simulink model "controller14"  (R2023a)
settings: Solver=FixedStepAuto  StartTime=0.0  StopTime=mdl.rt  RelTol=1e-3
values from neighbouring files (symbols this model uses):
  ctr = make_ext_tor_observer(rsim, mdl, ctr)    [step1_setup.m]
  ctr2 = ctr    [step1_setup.m]
  mdl = make_model(mdl,rsim)    [step1_setup.m]
  rbt = make_robot    [step1_setup.m]
  rbt2 = rbt    [step1_setup.m]
  som = make_somersault(mdl, rsim)    [step1_setup.m]
  traj = make_trajectory(ctr, mdl, rsim)    [step1_setup.m]
undefined symbols (not defined in the file or in its folder): archived_Eul_XYZ, archived_p_raw, DiscIntNeverNeededParam, lut, rsim, Standard_Devices, UDP_Protocol
libraries: simulink x27, dspfdesign x7, robotcorelib x6, sldrtlib x4, slrealtimeloglib x1, shared6dof x1, dspsrcs4 x1, uavutilslib x1
(part 2 of 3)

== system controller14/State filters/Subsystem1 ==
  p_dot : Inport
  data ready : Inport  Port=2
  Add1 : Sum  Inputs=+-
  Add2 : Sum  Inputs=+-
  Add3 : Sum  Commented=on  Inputs=+-
  Add4 : Sum  Inputs=+-
  Delay : Delay  Commented=on  DelayLength=1  InitialCondition=zeros(3,1)
  Delay1 : Delay  DelayLength=1  InitialCondition=zeros(3,1)
  Digital Filter Design2 : dspfdesign/Digital Filter Design  Commented=on  mwdsp_browser_bugfix_var=off
  Digital Clock : DigitalClock  SampleTime=mdl.T_high
  Gain : Gain  Commented=on  Gain=mdl.f_high
  Gain1 : Gain  Gain=mdl.f_high
  If : If  IfExpression=u1 == 0
  If Action Subsystem : Subsystem  TreatAsAtomicUnit=on
  If Action Subsystem1 : Subsystem  TreatAsAtomicUnit=on
  Merge : Merge
  Scope : Scope  Commented=on  NumInputPorts=2
  Triggered Subsystem : Subsystem  TreatAsAtomicUnit=on
  p_dotdot : Outport
  wires:
  data ready/1 -> Triggered Subsystem/Trigger
  Triggered Subsystem/1(Out1) -> Add1/1
  Triggered Subsystem/2(Output) -> Add1/2
  Triggered Subsystem/3(Output1) -> Add2/1
  Triggered Subsystem/4(Output2) -> Add2/2
  Add1/1 -> If Action Subsystem/1(In1)
  Add2/1 -> If Action Subsystem/2(In2), If/1
  If/2 -> If Action Subsystem/Action
  If/1 -> If Action Subsystem1/Action
  If Action Subsystem1/1(Out1) -> Merge/2
  If Action Subsystem/1(Out1) -> Merge/1
  Digital Clock/1 -> Triggered Subsystem/2(In2)
  Digital Filter Design2/1 -> Delay/1, Add3/1  "p_dot_filtered"
  Delay/1 -> Add3/2
  Add3/1 -> Gain/1
  Gain/1 -> Scope/2
  Add4/1 -> Gain1/1
  Delay1/1 -> Add4/2
  p_dot/1 -> Delay1/1, Add4/1, Digital Filter Design2/1, Triggered Subsystem/1(In1)  "p_dot_filtered"
  Gain1/1 -> p_dotdot/1, Scope/1

== system controller14/State filters/Subsystem4 ==
  In1 : Inport
  data ready : Inport  Port=2
  Add1 : Sum  Inputs=+-
  Add2 : Sum  Inputs=+-
  Digital Filter Design1 : dspfdesign/Digital Filter Design  mwdsp_browser_bugfix_var=off
  Digital Filter Design2 : dspfdesign/Digital Filter Design  Commented=on  mwdsp_browser_bugfix_var=off
  Digital Clock : DigitalClock  SampleTime=mdl.T_high
  If : If  IfExpression=u1 == 0
  If Action Subsystem : Subsystem  TreatAsAtomicUnit=on
  If Action Subsystem1 : Subsystem  TreatAsAtomicUnit=on
  Merge : Merge
  Scope : Scope  Commented=on  NumInputPorts=2
  Triggered Subsystem : Subsystem  TreatAsAtomicUnit=on
  p dot : Outport
  wires:
  In1/1 -> Triggered Subsystem/1(In1)
  data ready/1 -> Triggered Subsystem/Trigger
  Triggered Subsystem/1(Out1) -> Add1/1
  Triggered Subsystem/2(Output) -> Add1/2
  Triggered Subsystem/3(Output1) -> Add2/1
  Triggered Subsystem/4(Output2) -> Add2/2
  Add1/1 -> If Action Subsystem/1(In1)
  Add2/1 -> If Action Subsystem/2(In2), If/1
  If/2 -> If Action Subsystem/Action
  If/1 -> If Action Subsystem1/Action
  If Action Subsystem1/1(Out1) -> Merge/2
  If Action Subsystem/1(Out1) -> Merge/1
  Merge/1 -> Digital Filter Design1/1, Scope/1
  Digital Clock/1 -> Triggered Subsystem/2(In2)
  Digital Filter Design1/1 -> Scope/2, p dot/1  "p_dot_filtered"

== system controller14/State filters/Subsystem5 ==
  euler_angles : Inport
  data ready : Inport  Port=2
  sim enable : Inport  Port=3
  Add1 : Sum  Inputs=+-
  Add2 : Sum  Inputs=+-
  Add3 : Sum  Inputs=+-
  Delay : Delay  DelayLength=1  InitialCondition=zeros(9,1)
  Digital Clock : DigitalClock  SampleTime=1/10000
  Gain : Gain  Gain=400
  If : If  IfExpression=u1 == 0
  If Action Subsystem : Subsystem  TreatAsAtomicUnit=on
  If Action Subsystem1 : Subsystem  TreatAsAtomicUnit=on
  Merge : Merge
  Rotation Matrix : MATLAB Function  TreatAsAtomicUnit=on
  Rotation Matrix2 : MATLAB Function  TreatAsAtomicUnit=on
  Rotation Matrix3 : MATLAB Function  TreatAsAtomicUnit=on
  Switch1 : Switch  Criteria=u2 > Threshold  SaturateOnIntegerOverflow=off  InputSameDT=off
  Switch2 : Switch  Criteria=u2 > Threshold  SaturateOnIntegerOverflow=off  InputSameDT=off
  Triggered Subsystem : Subsystem  TreatAsAtomicUnit=on
  R : Outport
  Rdot : Outport  Port=2
  Omega : Outport  Port=3
  wires:
  Triggered Subsystem/1(Out1) -> Add1/1
  Triggered Subsystem/3(Output1) -> Add2/1
  Triggered Subsystem/4(Output2) -> Add2/2
  If Action Subsystem1/1(Out1) -> Merge/2
  If Action Subsystem/1(Out1) -> Merge/1
  Triggered Subsystem/2(Output) -> Add1/2
  Digital Clock/1 -> Triggered Subsystem/2(In2)
  data ready/1 -> Triggered Subsystem/Trigger
  Add2/1 -> If Action Subsystem/2(In2), If/1
  If/2 -> If Action Subsystem/Action
  If/1 -> If Action Subsystem1/Action
  Add1/1 -> If Action Subsystem/1(In1)
  euler_angles/1 -> Rotation Matrix/1(euler_angles)
  Rotation Matrix/1(R) -> Triggered Subsystem/1(R), R/1, Rotation Matrix3/1(R), Rotation Matrix2/1(R), Delay/1, Add3/1
  Delay/1 -> Add3/2
  Add3/1 -> Gain/1
  sim enable/1 -> Switch2/2, Switch1/2
  Gain/1 -> Switch2/1, Rotation Matrix2/2(Rdot)
  Rotation Matrix2/1(w) -> Switch1/1  "sim_omega"
  Merge/1 -> Switch2/3, Rotation Matrix3/2(Rdot)
  Rotation Matrix3/1(w) -> Switch1/3  "Vicon_omega"
  Switch1/1 -> Omega/1  "p_raw"
  Switch2/1 -> Rdot/1  "p_raw"

== system controller14/Subsystem/time ==
  constant : Constant
  time : DiscreteIntegrator  gainval=1  SampleTime=-1  UpperSaturationLimit=1  LowerSaturationLimit=0  ICPrevOutput=DiscIntNeverNeededParam  ICPrevScaledInput=DiscIntNeverNeededParam
  real times : Outport
  wires:
  constant/1 -> time/1
  time/1 -> real times/1

== system controller14/UDP send to Arduino/UDP send to Arduino DAC ==
  note: Aptinex DAC 20230818
  DAC1 : Inport
  DAC2 : Inport  Port=2
  DAC3 : Inport  Port=3
  DAC4 : Inport  Port=4
  DO2 : Inport  Port=5  OutDataTypeStr=boolean
  Bit Set : simulink/Logic and Bit Operations/Bit Set  iBit=12
  Demux : Demux
  Gain{,1..3} (4 alike) : Gain  Gain=4095/10  OutDataTypeStr=uint16
  Mux : Mux
  Mux1 : Mux
  Saturation : Saturate  UpperLimit=10  LowerLimit=0
  Switch : Switch  Criteria=u2 ~= 0  OutDataTypeStr=uint16  SaturateOnIntegerOverflow=off  InputSameDT=off
  Output : Outport
  wires:
  Gain3/1 -> Mux1/4  "UDP uint16 4"
  Gain1/1 -> Mux1/2  "UDP uint16 2"
  Gain/1 -> Bit Set/1, Switch/3  "UDP uint16 1"
  Gain2/1 -> Mux1/3  "UDP uint16 3"
  DO2/1 -> Switch/2
  Bit Set/1 -> Switch/1
  Mux1/1 -> Output/1
  Switch/1 -> Mux1/1
  Demux/1 -> Gain/1
  Demux/2 -> Gain1/1
  Demux/3 -> Gain2/1
  Demux/4 -> Gain3/1
  DAC1/1 -> Mux/1  "DAC voltage 1"
  DAC2/1 -> Mux/2  "DAC voltage 2"
  DAC3/1 -> Mux/3  "DAC voltage 3"
  DAC4/1 -> Mux/4  "DAC voltage 4"
  Mux/1 -> Saturation/1
  Saturation/1 -> Demux/1

== system controller14/signal generator1/Bias_Signal ==
  note: time constant = 0.002sec
  QuasiEnable : Inport
  BiasVolts : Inport  Port=2
  AveragedBias : Subsystem
  PreGain : Gain
  Product : Product  RndMeth=Zero
  SIgnalForRamp_binary : Subsystem
  SaturatingRamp : DiscreteIntegrator  gainval=100  SampleTime=-1  LimitOutput=on  UpperSaturationLimit=1  LowerSaturationLimit=0  ICPrevOutput=DiscIntNeverNeededParam  ICPrevScaledInput=DiscIntNeverNeededParam
  BiasD2A : Outport
  wires:
  PreGain/1 -> BiasD2A/1
  BiasVolts/1 -> AveragedBias/1(In1)
  QuasiEnable/1 -> SIgnalForRamp_binary/1(In1)
  SIgnalForRamp_binary/1(Out1) -> SaturatingRamp/1
  SaturatingRamp/1 -> Product/1
  AveragedBias/1(Out1) -> Product/2
  Product/1 -> PreGain/1

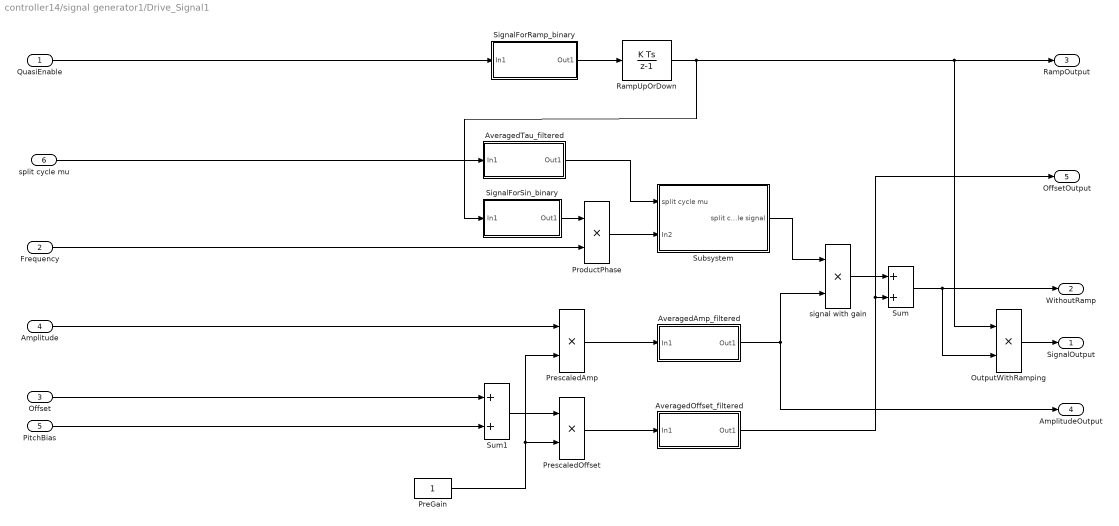
== system controller14/signal generator1/Drive_Signal1 ==
  QuasiEnable : Inport
  Frequency : Inport  Port=2
  Offset : Inport  Port=3
  Amplitude : Inport  Port=4
  PitchBias : Inport  Port=5
  split cycle mu : Inport  Port=6
  AveragedAmp_filtered : Subsystem
  AveragedOffset_filtered : Subsystem
  AveragedTau_filtered : Subsystem
  OutputWithRamping : Product  RndMeth=Zero
  PreGain : Constant
  PrescaledAmp : Product  RndMeth=Zero
  PrescaledOffset : Product  RndMeth=Zero
  ProductPhase : Product  RndMeth=Zero
  RampUpOrDown : DiscreteIntegrator  gainval=100  SampleTime=-1  LimitOutput=on  UpperSaturationLimit=1  LowerSaturationLimit=0  ICPrevOutput=DiscIntNeverNeededParam  ICPrevScaledInput=DiscIntNeverNeededParam
  SignalForRamp_binary : Subsystem
  SignalForSin_binary : Subsystem
  Subsystem : Subsystem
  Sum : Sum
  Sum1 : Sum
  signal with gain : Product  RndMeth=Zero
  SignalOutput : Outport
  WithoutRamp : Outport  Port=2
  RampOutput : Outport  Port=3
  AmplitudeOutput : Outport  Port=4
  OffsetOutput : Outport  Port=5
  wires:
  PrescaledAmp/1 -> AveragedAmp_filtered/1(In1)
  Sum/1 -> OutputWithRamping/2, WithoutRamp/1
  RampUpOrDown/1 -> RampOutput/1, OutputWithRamping/1, SignalForSin_binary/1(In1)
  QuasiEnable/1 -> SignalForRamp_binary/1(In1)
  SignalForRamp_binary/1(Out1) -> RampUpOrDown/1
  Amplitude/1 -> PrescaledAmp/1
  signal with gain/1 -> Sum/1
  Frequency/1 -> ProductPhase/2
  SignalForSin_binary/1(Out1) -> ProductPhase/1
  ProductPhase/1 -> Subsystem/2(In2)
  AveragedOffset_filtered/1(Out1) -> Sum/2, OffsetOutput/1
  PrescaledOffset/1 -> AveragedOffset_filtered/1(In1)
  PreGain/1 -> PrescaledAmp/2, PrescaledOffset/2
  OutputWithRamping/1 -> SignalOutput/1
  AveragedAmp_filtered/1(Out1) -> signal with gain/2, AmplitudeOutput/1
  Sum1/1 -> PrescaledOffset/1
  Offset/1 -> Sum1/1
  PitchBias/1 -> Sum1/2
  AveragedTau_filtered/1(Out1) -> Subsystem/1(split cycle mu)
  split cycle mu/1 -> AveragedTau_filtered/1(In1)
  Subsystem/1(split cycle signal) -> signal with gain/1

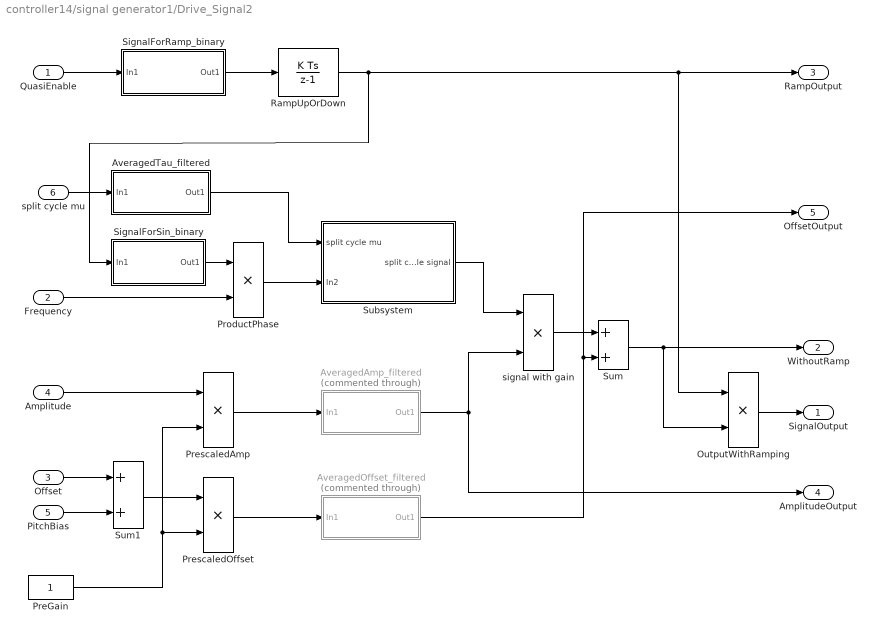
== system controller14/signal generator1/Drive_Signal2 ==
  QuasiEnable : Inport
  Frequency : Inport  Port=2
  Offset : Inport  Port=3
  Amplitude : Inport  Port=4
  PitchBias : Inport  Port=5
  split cycle mu : Inport  Port=6
  AveragedAmp_filtered : Subsystem  Commented=through
  AveragedOffset_filtered : Subsystem  Commented=through
  AveragedTau_filtered : Subsystem
  OutputWithRamping : Product  RndMeth=Zero
  PreGain : Constant
  PrescaledAmp : Product  RndMeth=Zero
  PrescaledOffset : Product  RndMeth=Zero
  ProductPhase : Product  RndMeth=Zero
  RampUpOrDown : DiscreteIntegrator  gainval=100  SampleTime=-1  LimitOutput=on  UpperSaturationLimit=1  LowerSaturationLimit=0  ICPrevOutput=DiscIntNeverNeededParam  ICPrevScaledInput=DiscIntNeverNeededParam
  SignalForRamp_binary : Subsystem
  SignalForSin_binary : Subsystem
  Subsystem : Subsystem
  Sum : Sum
  Sum1 : Sum
  signal with gain : Product  RndMeth=Zero
  SignalOutput : Outport
  WithoutRamp : Outport  Port=2
  RampOutput : Outport  Port=3
  AmplitudeOutput : Outport  Port=4
  OffsetOutput : Outport  Port=5
  wires:
  PrescaledAmp/1 -> AveragedAmp_filtered/1(In1)
  Sum/1 -> OutputWithRamping/2, WithoutRamp/1
  RampUpOrDown/1 -> RampOutput/1, OutputWithRamping/1, SignalForSin_binary/1(In1)
  QuasiEnable/1 -> SignalForRamp_binary/1(In1)
  SignalForRamp_binary/1(Out1) -> RampUpOrDown/1
  Amplitude/1 -> PrescaledAmp/1
  signal with gain/1 -> Sum/1
  Frequency/1 -> ProductPhase/2
  SignalForSin_binary/1(Out1) -> ProductPhase/1
  ProductPhase/1 -> Subsystem/2(In2)
  AveragedOffset_filtered/1(Out1) -> Sum/2, OffsetOutput/1
  PrescaledOffset/1 -> AveragedOffset_filtered/1(In1)
  PreGain/1 -> PrescaledAmp/2, PrescaledOffset/2
  OutputWithRamping/1 -> SignalOutput/1
  AveragedAmp_filtered/1(Out1) -> signal with gain/2, AmplitudeOutput/1
  Sum1/1 -> PrescaledOffset/1
  Offset/1 -> Sum1/1
  PitchBias/1 -> Sum1/2
  AveragedTau_filtered/1(Out1) -> Subsystem/1(split cycle mu)
  split cycle mu/1 -> AveragedTau_filtered/1(In1)
  Subsystem/1(split cycle signal) -> signal with gain/1

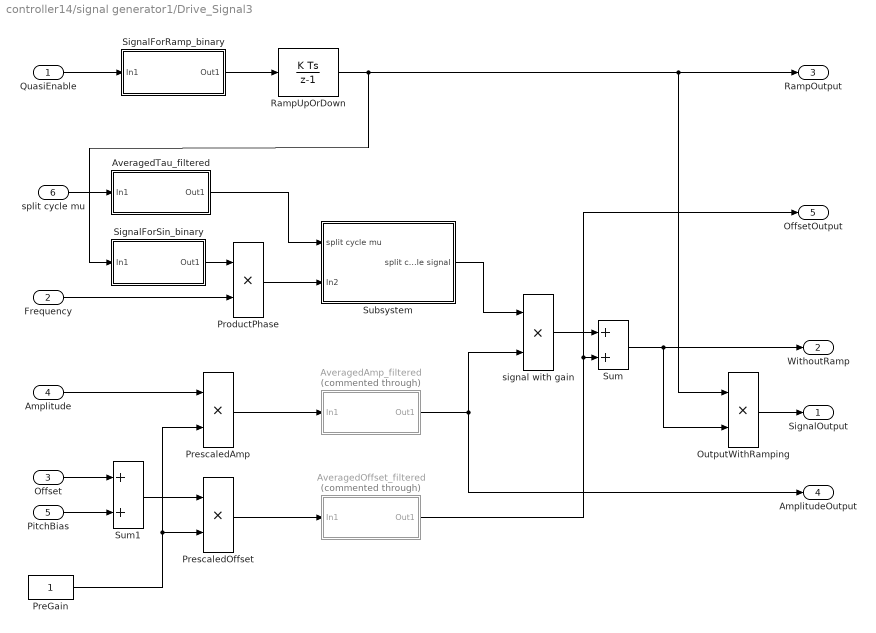
== system controller14/signal generator1/Drive_Signal3 ==
  QuasiEnable : Inport
  Frequency : Inport  Port=2
  Offset : Inport  Port=3
  Amplitude : Inport  Port=4
  PitchBias : Inport  Port=5
  split cycle mu : Inport  Port=6
  AveragedAmp_filtered : Subsystem  Commented=through
  AveragedOffset_filtered : Subsystem  Commented=through
  AveragedTau_filtered : Subsystem
  OutputWithRamping : Product  RndMeth=Zero
  PreGain : Constant
  PrescaledAmp : Product  RndMeth=Zero
  PrescaledOffset : Product  RndMeth=Zero
  ProductPhase : Product  RndMeth=Zero
  RampUpOrDown : DiscreteIntegrator  gainval=100  SampleTime=-1  LimitOutput=on  UpperSaturationLimit=1  LowerSaturationLimit=0  ICPrevOutput=DiscIntNeverNeededParam  ICPrevScaledInput=DiscIntNeverNeededParam
  SignalForRamp_binary : Subsystem
  SignalForSin_binary : Subsystem
  Subsystem : Subsystem
  Sum : Sum
  Sum1 : Sum
  signal with gain : Product  RndMeth=Zero
  SignalOutput : Outport
  WithoutRamp : Outport  Port=2
  RampOutput : Outport  Port=3
  AmplitudeOutput : Outport  Port=4
  OffsetOutput : Outport  Port=5
  wires:
  PrescaledAmp/1 -> AveragedAmp_filtered/1(In1)
  Sum/1 -> OutputWithRamping/2, WithoutRamp/1
  RampUpOrDown/1 -> RampOutput/1, OutputWithRamping/1, SignalForSin_binary/1(In1)
  QuasiEnable/1 -> SignalForRamp_binary/1(In1)
  SignalForRamp_binary/1(Out1) -> RampUpOrDown/1
  Amplitude/1 -> PrescaledAmp/1
  signal with gain/1 -> Sum/1
  Frequency/1 -> ProductPhase/2
  SignalForSin_binary/1(Out1) -> ProductPhase/1
  ProductPhase/1 -> Subsystem/2(In2)
  AveragedOffset_filtered/1(Out1) -> Sum/2, OffsetOutput/1
  PrescaledOffset/1 -> AveragedOffset_filtered/1(In1)
  PreGain/1 -> PrescaledAmp/2, PrescaledOffset/2
  OutputWithRamping/1 -> SignalOutput/1
  AveragedAmp_filtered/1(Out1) -> signal with gain/2, AmplitudeOutput/1
  Sum1/1 -> PrescaledOffset/1
  Offset/1 -> Sum1/1
  PitchBias/1 -> Sum1/2
  AveragedTau_filtered/1(Out1) -> Subsystem/1(split cycle mu)
  split cycle mu/1 -> AveragedTau_filtered/1(In1)
  Subsystem/1(split cycle signal) -> signal with gain/1

== system controller14/signal generator1/Drive_Signal4 ==
  QuasiEnable : Inport
  Frequency : Inport  Port=2
  Offset : Inport  Port=3
  Amplitude : Inport  Port=4
  PitchBias : Inport  Port=5
  split cycle mu : Inport  Port=6
  AveragedAmp_filtered : Subsystem
  AveragedOffset_filtered : Subsystem
  AveragedTau_filtered : Subsystem
  OutputWithRamping : Product  RndMeth=Zero
  PreGain : Constant
  PrescaledAmp : Product  RndMeth=Zero
  PrescaledOffset : Product  RndMeth=Zero
  ProductPhase : Product  RndMeth=Zero
  RampUpOrDown : DiscreteIntegrator  gainval=100  SampleTime=-1  LimitOutput=on  UpperSaturationLimit=1  LowerSaturationLimit=0  ICPrevOutput=DiscIntNeverNeededParam  ICPrevScaledInput=DiscIntNeverNeededParam
  SignalForRamp_binary : Subsystem
  SignalForSin_binary : Subsystem
  Subsystem : Subsystem
  Sum : Sum
  Sum1 : Sum
  signal with gain : Product  RndMeth=Zero
  SignalOutput : Outport
  WithoutRamp : Outport  Port=2
  RampOutput : Outport  Port=3
  AmplitudeOutput : Outport  Port=4
  OffsetOutput : Outport  Port=5
  wires:
  PrescaledAmp/1 -> AveragedAmp_filtered/1(In1)
  Sum/1 -> OutputWithRamping/2, WithoutRamp/1
  RampUpOrDown/1 -> RampOutput/1, OutputWithRamping/1, SignalForSin_binary/1(In1)
  QuasiEnable/1 -> SignalForRamp_binary/1(In1)
  SignalForRamp_binary/1(Out1) -> RampUpOrDown/1
  Amplitude/1 -> PrescaledAmp/1
  signal with gain/1 -> Sum/1
  Frequency/1 -> ProductPhase/2
  SignalForSin_binary/1(Out1) -> ProductPhase/1
  ProductPhase/1 -> Subsystem/2(In2)
  AveragedOffset_filtered/1(Out1) -> Sum/2, OffsetOutput/1
  PrescaledOffset/1 -> AveragedOffset_filtered/1(In1)
  PreGain/1 -> PrescaledAmp/2, PrescaledOffset/2
  OutputWithRamping/1 -> SignalOutput/1
  AveragedAmp_filtered/1(Out1) -> signal with gain/2, AmplitudeOutput/1
  Sum1/1 -> PrescaledOffset/1
  Offset/1 -> Sum1/1
  PitchBias/1 -> Sum1/2
  AveragedTau_filtered/1(Out1) -> Subsystem/1(split cycle mu)
  split cycle mu/1 -> AveragedTau_filtered/1(In1)
  Subsystem/1(split cycle signal) -> signal with gain/1

== system controller14/signal generator1/SignalSaturationLimit ==
  BiasMax : Inport
  SignalRaw : Inport  Port=2
  GainBias : Gain
  MaxOf : MinMax  Function=max  Inputs=2
  MinOf : MinMax  Inputs=2
  ground : Constant
  SignalSatd : Outport
  wires:
  BiasMax/1 -> GainBias/1
  SignalRaw/1 -> MinOf/2
  MinOf/1 -> MaxOf/1
  MaxOf/1 -> SignalSatd/1
  GainBias/1 -> MinOf/1
  ground/1 -> MaxOf/2

== system controller14/signal generator1/SignalSaturationLimit1 ==
  BiasMax : Inport
  SignalRaw : Inport  Port=2
  GainBias : Gain
  MaxOf : MinMax  Function=max  Inputs=2
  MinOf : MinMax  Inputs=2
  ground : Constant
  SignalSatd : Outport
  wires:
  BiasMax/1 -> GainBias/1
  SignalRaw/1 -> MinOf/2
  MinOf/1 -> MaxOf/1
  MaxOf/1 -> SignalSatd/1
  GainBias/1 -> MinOf/1
  ground/1 -> MaxOf/2

== system controller14/signal generator1/SignalSaturationLimit2 ==
  BiasMax : Inport
  SignalRaw : Inport  Port=2
  GainBias : Gain
  MaxOf : MinMax  Function=max  Inputs=2
  MinOf : MinMax  Inputs=2
  ground : Constant
  SignalSatd : Outport
  wires:
  BiasMax/1 -> GainBias/1
  SignalRaw/1 -> MinOf/2
  MinOf/1 -> MaxOf/1
  MaxOf/1 -> SignalSatd/1
  GainBias/1 -> MinOf/1
  ground/1 -> MaxOf/2

== system controller14/signal generator1/SignalSaturationLimit3 ==
  BiasMax : Inport
  SignalRaw : Inport  Port=2
  GainBias : Gain
  MaxOf : MinMax  Function=max  Inputs=2
  MinOf : MinMax  Inputs=2
  ground : Constant
  SignalSatd : Outport
  wires:
  BiasMax/1 -> GainBias/1
  SignalRaw/1 -> MinOf/2
  MinOf/1 -> MaxOf/1
  MaxOf/1 -> SignalSatd/1
  GainBias/1 -> MinOf/1
  ground/1 -> MaxOf/2

== system controller14/signal generator1/signal generator 1 ==
  quasi enable : Inport
  max voltage : Inport  Port=2
  frequency : Inport  Port=3
  half amplitude : Inport  Port=4
  2pi : Gain  Gain=2*pi
  Add1 : Sum
  Add2 : Sum
  Gain1 : Gain  Gain=-1
  OutputWithRamping : Product  RndMeth=Zero
  RampUpOrDown : DiscreteIntegrator  gainval=100  SampleTime=-1  LimitOutput=on  UpperSaturationLimit=1  LowerSaturationLimit=0  ICPrevOutput=DiscIntNeverNeededParam  ICPrevScaledInput=DiscIntNeverNeededParam
  Scope1 : Scope  Commented=on
  Scope2 : Scope  Commented=on
  SignalForRamp_binary : Subsystem
  SignalSaturationLimit4 : Subsystem
  Subsystem : Subsystem
  deg to rad : Gain  Gain=pi/180
  first harmonic : Trigonometry  Operator=cos  OutputSignalType=real
  get max voltage : Subsystem
  omega*t : DiscreteIntegrator  SampleTime=-1  ICPrevOutput=DiscIntNeverNeededParam  ICPrevScaledInput=DiscIntNeverNeededParam
  phase offset : Constant  Value=180
  signal with gain1 : Product  RndMeth=Zero
  SignalSatd : Outport
  wires:
  first harmonic/1 -> Gain1/1
  Subsystem/1(output) -> Add2/2, signal with gain1/2
  RampUpOrDown/1 -> OutputWithRamping/1
  deg to rad/1 -> Add1/1
  Add1/1 -> first harmonic/1
  max voltage/1 -> get max voltage/2(max voltage)
  2pi/1 -> omega*t/1
  signal with gain1/1 -> Add2/1
  Add2/1 -> OutputWithRamping/2
  omega*t/1 -> Add1/2
  Gain1/1 -> Subsystem/1(cos wave), signal with gain1/1
  quasi enable/1 -> Scope2/1, SignalForRamp_binary/1(EnableSignal), get max voltage/1(QuasiEnable)
  SignalForRamp_binary/1(Out1) -> RampUpOrDown/1
  phase offset/1 -> deg to rad/1
  OutputWithRamping/1 -> SignalSaturationLimit4/2(SignalRaw)
  get max voltage/1(max signa;) -> Scope1/1, SignalSaturationLimit4/1(Max)
  SignalSaturationLimit4/1(SignalSatd) -> SignalSatd/1
  half amplitude/1 -> Subsystem/2(new_amplitude)
  frequency/1 -> 2pi/1

== system controller14/signal generator1/signal generator 2 ==
  quasi enable : Inport
  max voltage : Inport  Port=2
  frequency : Inport  Port=3
  half amplitude : Inport  Port=4
  2pi : Gain  Gain=2*pi
  Add1 : Sum
  Add2 : Sum
  Gain1 : Gain  Gain=-1
  OutputWithRamping : Product  RndMeth=Zero
  RampUpOrDown : DiscreteIntegrator  gainval=100  SampleTime=-1  LimitOutput=on  UpperSaturationLimit=1  LowerSaturationLimit=0  ICPrevOutput=DiscIntNeverNeededParam  ICPrevScaledInput=DiscIntNeverNeededParam
  SignalForRamp_binary : Subsystem
  SignalSaturationLimit4 : Subsystem
  Subsystem : Subsystem
  deg to rad : Gain  Gain=pi/180
  first harmonic : Trigonometry  Operator=cos  OutputSignalType=real
  get max voltage : Subsystem
  omega*t : DiscreteIntegrator  SampleTime=-1  ICPrevOutput=DiscIntNeverNeededParam  ICPrevScaledInput=DiscIntNeverNeededParam
  phase offset : Constant  Value=0
  signal with gain1 : Product  RndMeth=Zero
  SignalSatd : Outport
  wires:
  first harmonic/1 -> Gain1/1
  Subsystem/1(output) -> Add2/2, signal with gain1/2
  RampUpOrDown/1 -> OutputWithRamping/1
  deg to rad/1 -> Add1/1
  Add1/1 -> first harmonic/1
  max voltage/1 -> get max voltage/2(max voltage)
  2pi/1 -> omega*t/1
  signal with gain1/1 -> Add2/1
  Add2/1 -> OutputWithRamping/2
  omega*t/1 -> Add1/2
  Gain1/1 -> Subsystem/1(cos wave), signal with gain1/1
  quasi enable/1 -> SignalForRamp_binary/1(EnableSignal), get max voltage/1(QuasiEnable)
  SignalForRamp_binary/1(Out1) -> RampUpOrDown/1
  phase offset/1 -> deg to rad/1
  OutputWithRamping/1 -> SignalSaturationLimit4/2(SignalRaw)
  get max voltage/1(max signa;) -> SignalSaturationLimit4/1(Max)
  SignalSaturationLimit4/1(SignalSatd) -> SignalSatd/1
  half amplitude/1 -> Subsystem/2(new_amplitude)
  frequency/1 -> 2pi/1

== system controller14/signal generator1/signal generator 3 ==
  quasi enable : Inport
  max voltage : Inport  Port=2
  frequency : Inport  Port=3
  half amplitude : Inport  Port=4
  2pi : Gain  Gain=2*pi
  Add1 : Sum
  Add2 : Sum
  Gain1 : Gain  Gain=-1
  OutputWithRamping : Product  RndMeth=Zero
  RampUpOrDown : DiscreteIntegrator  gainval=100  SampleTime=-1  LimitOutput=on  UpperSaturationLimit=1  LowerSaturationLimit=0  ICPrevOutput=DiscIntNeverNeededParam  ICPrevScaledInput=DiscIntNeverNeededParam
  SignalForRamp_binary : Subsystem
  SignalSaturationLimit4 : Subsystem
  Subsystem : Subsystem
  deg to rad : Gain  Gain=pi/180
  first harmonic : Trigonometry  Operator=cos  OutputSignalType=real
  get max voltage : Subsystem
  omega*t : DiscreteIntegrator  SampleTime=-1  ICPrevOutput=DiscIntNeverNeededParam  ICPrevScaledInput=DiscIntNeverNeededParam
  phase offset : Constant  Value=180
  signal with gain1 : Product  RndMeth=Zero
  SignalSatd : Outport
  wires:
  first harmonic/1 -> Gain1/1
  RampUpOrDown/1 -> OutputWithRamping/1
  deg to rad/1 -> Add1/1
  Add1/1 -> first harmonic/1
  max voltage/1 -> get max voltage/2(max voltage)
  2pi/1 -> omega*t/1
  signal with gain1/1 -> Add2/1
  Add2/1 -> OutputWithRamping/2
  omega*t/1 -> Add1/2
  Gain1/1 -> Subsystem/1(cos wave), signal with gain1/1
  quasi enable/1 -> SignalForRamp_binary/1(EnableSignal), get max voltage/1(QuasiEnable)
  SignalForRamp_binary/1(Out1) -> RampUpOrDown/1
  phase offset/1 -> deg to rad/1
  OutputWithRamping/1 -> SignalSaturationLimit4/2(SignalRaw)
  get max voltage/1(max signa;) -> SignalSaturationLimit4/1(Max)
  SignalSaturationLimit4/1(SignalSatd) -> SignalSatd/1
  frequency/1 -> 2pi/1
  half amplitude/1 -> Subsystem/2(new_amplitude)
  Subsystem/1(output) -> Add2/2, signal with gain1/2

== system controller14/signal generator1/signal generator 4 ==
  quasi enable : Inport
  max voltage : Inport  Port=2
  frequency : Inport  Port=3
  half amplitude : Inport  Port=4
  2pi : Gain  Gain=2*pi
  Add1 : Sum
  Add2 : Sum
  Gain1 : Gain  Gain=-1
  OutputWithRamping : Product  RndMeth=Zero
  RampUpOrDown : DiscreteIntegrator  gainval=100  SampleTime=-1  LimitOutput=on  UpperSaturationLimit=1  LowerSaturationLimit=0  ICPrevOutput=DiscIntNeverNeededParam  ICPrevScaledInput=DiscIntNeverNeededParam
  SignalForRamp_binary : Subsystem
  SignalSaturationLimit4 : Subsystem
  Subsystem : Subsystem
  deg to rad : Gain  Gain=pi/180
  first harmonic : Trigonometry  Operator=cos  OutputSignalType=real
  get max voltage : Subsystem
  omega*t : DiscreteIntegrator  SampleTime=-1  ICPrevOutput=DiscIntNeverNeededParam  ICPrevScaledInput=DiscIntNeverNeededParam
  phase offset : Constant  Value=0
  signal with gain1 : Product  RndMeth=Zero
  SignalSatd : Outport
  wires:
  first harmonic/1 -> Gain1/1
  RampUpOrDown/1 -> OutputWithRamping/1
  deg to rad/1 -> Add1/1
  Add1/1 -> first harmonic/1
  max voltage/1 -> get max voltage/2(max voltage)
  2pi/1 -> omega*t/1
  signal with gain1/1 -> Add2/1
  Add2/1 -> OutputWithRamping/2
  omega*t/1 -> Add1/2
  Gain1/1 -> signal with gain1/1, Subsystem/1(cos wave)
  quasi enable/1 -> SignalForRamp_binary/1(EnableSignal), get max voltage/1(QuasiEnable)
  SignalForRamp_binary/1(Out1) -> RampUpOrDown/1
  phase offset/1 -> deg to rad/1
  OutputWithRamping/1 -> SignalSaturationLimit4/2(SignalRaw)
  get max voltage/1(max signa;) -> SignalSaturationLimit4/1(Max)
  SignalSaturationLimit4/1(SignalSatd) -> SignalSatd/1
  half amplitude/1 -> Subsystem/2(new_amplitude)
  frequency/1 -> 2pi/1
  Subsystem/1(output) -> signal with gain1/2, Add2/2

== system controller14/Control scheme/attitude and thrust controller/Subsystem ==
  att_e : Inport
  alt_e : Inport  Port=2
  Delay2 : Delay  DelayLength=1  InitialCondition=zeros(4,1)
  Digital Clock : DigitalClock  SampleTime=mdl.T
  Discrete-Time Integrator : DiscreteIntegrator  InitialCondition=zeros(4,1)  SampleTime=mdl.T  LimitOutput=on  UpperSaturationLimit=ctr.integral.lim.upper  LowerSaturationLimit=ctr.integral.lim.lower  ICPrevOutput=DiscIntNeverNeededParam  ICPrevScaledInput=DiscIntNeverNeededParam
  Gain : Gain  Gain=ctr.gain.ati
  Gain1 : Gain  Gain=ctr.gain.ali
  MATLAB Function : MATLAB Function  TreatAsAtomicUnit=on
  Mux : Mux  Inputs=2
  Product : Product
  Selector : Selector  InputPortWidth=4  IndexOptions=Index vector (dialog)  Indices=[1 2 3]  OutputSizes=1
  Selector1 : Selector  InputPortWidth=4  IndexOptions=Index vector (dialog)  Indices=[4]  OutputSizes=1
  int thrust : Scope
  int torque : Scope
  Out1 : Outport
  wires:
  Digital Clock/1 -> MATLAB Function/1(time)
  MATLAB Function/1(en_int) -> Product/1
  Mux/1 -> Product/2
  Discrete-Time Integrator/1 -> Delay2/1
  Selector1/1 -> int thrust/1  "int thrust acc"
  Delay2/1 -> Selector1/1, Selector/1, Out1/1
  Gain/1 -> Mux/1
  att_e/1 -> Gain/1
  Product/1 -> Discrete-Time Integrator/1
  Selector/1 -> int torque/1  "int torque"
  Gain1/1 -> Mux/2
  alt_e/1 -> Gain1/1

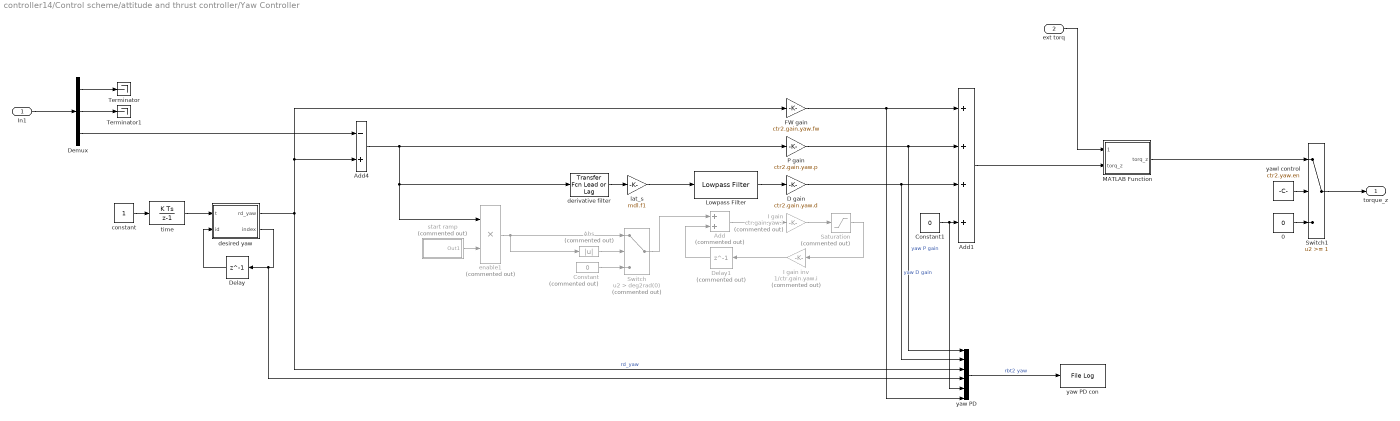
== system controller14/Control scheme/attitude and thrust controller/Yaw Controller ==
  In1 : Inport
  ext torq : Inport  Port=2
  0 : Constant  Value=0  SampleTime=-1
  Abs : Abs  Commented=on  SaturateOnIntegerOverflow=off
  Add : Sum  Commented=on
  Add1 : Sum  Inputs=++++
  Add4 : Sum  Inputs=-+
  Constant : Constant  Commented=on  Value=0
  Constant1 : Constant  Value=0  SampleTime=-1
  D gain : Gain  Gain=ctr2.gain.yaw.d
  Delay : Delay  DelayLength=1  InitialCondition=1
  Delay1 : Delay  Commented=on  DelayLength=1
  Demux : Demux  Outputs=3
  FW gain : Gain  Gain=ctr2.gain.yaw.fw
  I gain : Gain  Commented=on  Gain=ctr.gain.yaw.i
  I gain inv : Gain  Commented=on  Gain=1/ctr.gain.yaw.i
  Lowpass Filter : dspfdesign/Lowpass Filter  FilterType=FIR  DesignForMinimumOrder=on  FilterOrder=2000  PassbandFrequency=7  StopbandFrequency=90  PassbandRipple=0.5  StopbandAttenuation=75  SampleRateMode=Specify on dialog  SampleRate=10000  SimulateUsing=Interpreted execution  roundingMode=Floor  coeffsDataTypeStr=fixdt(1,16)
  MATLAB Function : MATLAB Function  TreatAsAtomicUnit=on
  P gain : Gain  Gain=ctr2.gain.yaw.p
  Saturation : Saturate  Commented=on  UpperLimit=ctr.integral.yaw.upper  LowerLimit=ctr.integral.yaw.lower
  Switch : Switch  Commented=on  Criteria=u2 > Threshold  Threshold=deg2rad(0)  SaturateOnIntegerOverflow=off  InputSameDT=off
  Switch1 : Switch  Threshold=1  SaturateOnIntegerOverflow=off  InputSameDT=off
  Terminator : Terminator
  Terminator1 : Terminator
  constant : Constant
  derivative filter : simulink/Discrete/Transfer Fcn Lead or Lag  PoleZ=mdl.zf1  ZeroZ=1  ICPrevOutput=0.0  ICPrevInput=0.0  DoSatur=off
  desired yaw : MATLAB Function  TreatAsAtomicUnit=on
  enable1 : Product  Commented=on  Inputs=**
  lat_s : Gain  Gain=mdl.f1
  start ramp : Subsystem  Commented=on
  time : DiscreteIntegrator  gainval=1  SampleTime=-1  UpperSaturationLimit=1  LowerSaturationLimit=0  ICPrevOutput=DiscIntNeverNeededParam  ICPrevScaledInput=DiscIntNeverNeededParam
  yaw PD : Mux  Inputs=6
  yaw PD con : slrealtimeloglib/File Log  decimation=1  inputProcessing=Elements as channels (sample based)
  yawl control : Constant  Value=ctr2.yaw.en
  torque_z : Outport
  wires:
  Demux/1 -> Terminator/1
  Demux/2 -> Terminator1/1
  Demux/3 -> Add4/1
  0/1 -> Switch1/3
  yawl control/1 -> Switch1/2
  In1/1 -> Demux/1
  Add4/1 -> P gain/1, enable1/1, derivative filter/1
  Switch1/1 -> torque_z/1
  derivative filter/1 -> lat_s/1
  Add1/1 -> MATLAB Function/2("torq_z ")
  P gain/1 -> yaw PD/1, Add1/2  "yaw P gain"
  D gain/1 -> yaw PD/2, Add1/3  "yaw D gain"
  yaw PD/1 -> yaw PD con/1  "rbt2 yaw"
  Lowpass Filter/1 -> D gain/1
  lat_s/1 -> Lowpass Filter/1
  constant/1 -> time/1
  time/1 -> desired yaw/1(t)
  desired yaw/1(rd_yaw) -> FW gain/1, Add4/2, yaw PD/3  "rd_yaw"
  desired yaw/2(index) -> yaw PD/4, Delay/1
  Delay/1 -> desired yaw/2(id)
  Saturation/1 -> I gain inv/1
  I gain/1 -> Saturation/1
  enable1/1 -> Switch/1, Abs/1
  Delay1/1 -> Add/2
  Add/1 -> I gain/1
  I gain inv/1 -> Delay1/1
  start ramp/1(Out1) -> enable1/2
  Constant/1 -> Switch/3
  Switch/1 -> Add/1
  Abs/1 -> Switch/2
  FW gain/1 -> yaw PD/6, Add1/1
  Constant1/1 -> yaw PD/5, Add1/4
  MATLAB Function/1(torq_z) -> Switch1/1
  ext torq/1 -> MATLAB Function/1(torq_ext)

== system controller14/Control scheme/attitude and thrust controller/time ==
  constant : Constant
  time : DiscreteIntegrator  gainval=1  SampleTime=-1  UpperSaturationLimit=1  LowerSaturationLimit=0  ICPrevOutput=DiscIntNeverNeededParam  ICPrevScaledInput=DiscIntNeverNeededParam
  real times : Outport
  wires:
  constant/1 -> time/1
  time/1 -> real times/1

== system controller14/Control scheme/observer/Rotaion ==
  Euler : Inport
  Rotation Matrix : MATLAB Function  TreatAsAtomicUnit=on
  Rotation Matrix1 : MATLAB Function  TreatAsAtomicUnit=on
  filtered derivative : Subsystem
  R : Outport
  Rdot : Outport  Port=2
  Omega : Outport  Port=3
  wires:
  Rotation Matrix/1(R) -> filtered derivative/1(In1), Rotation Matrix1/1(R), R/1
  Euler/1 -> Rotation Matrix/1(euler_angles)
  filtered derivative/1(Out1) -> Rotation Matrix1/2(Rdot), Rdot/1
  Rotation Matrix1/1(w) -> Omega/1

== system controller14/Control scheme/observer/lateral observer ==
  XYZ : Inport
  derivative filter : simulink/Discrete/Transfer Fcn Lead or Lag  PoleZ=mdl.zf1  ZeroZ=1  ICPrevOutput=0.0  ICPrevInput=0.0  DoSatur=off
  derivative filter1 : simulink/Discrete/Transfer Fcn Lead or Lag  PoleZ=mdl.zf2  ZeroZ=1  ICPrevOutput=0.0  ICPrevInput=0.0  DoSatur=off
  derivative filter2 : simulink/Discrete/Transfer Fcn Lead or Lag  PoleZ=mdl.zf2  ZeroZ=1  ICPrevOutput=0.0  ICPrevInput=0.0  DoSatur=off
  lat_s : Gain  Gain=mdl.f1
  lat_s2 : Gain  Gain=mdl.f2
  lat_s2_ : Gain  Gain=mdl.f2
  saturation : Subsystem
  r : Outport
  r_dot : Outport  Port=2
  r_dotdot : Outport  Port=3
  wires:
  derivative filter1/1 -> derivative filter2/1
  derivative filter/1 -> lat_s/1
  XYZ/1 -> derivative filter/1, derivative filter1/1, r/1
  derivative filter2/1 -> lat_s2/1
  lat_s/1 -> r_dot/1
  lat_s2/1 -> lat_s2_/1
  lat_s2_/1 -> saturation/1(In1)
  saturation/1(Out1) -> r_dotdot/1

== system controller14/State filters/Subsystem1/If Action Subsystem ==
  In1 : Inport
  In2 : Inport  Port=2
  Action Port : ActionPort  ActionPortLabel=else
  Divide : Product  Inputs=*/
  Out1 : Outport
  wires:
  In1/1 -> Divide/1
  In2/1 -> Divide/2
  Divide/1 -> Out1/1

== system controller14/State filters/Subsystem1/If Action Subsystem1 ==
  Action Port : ActionPort  ActionPortLabel=if(u1 == 0)
  Constant : Constant  Value=[0;0;0]
  Out1 : Outport
  wires:
  Constant/1 -> Out1/1

== system controller14/State filters/Subsystem1/Triggered Subsystem ==
  In1 : Inport
  In2 : Inport  Port=2
  Trigger : TriggerPort  VariantControl=(inherit)
  Scope : Scope  Commented=on  NumInputPorts=2
  Unit Delay : UnitDelay  SampleTime=-1  HasFrameUpgradeWarning=on
  Unit Delay1 : UnitDelay  SampleTime=-1  HasFrameUpgradeWarning=on
  Out1 : Outport
  Output : Outport  Port=2
  Output1 : Outport  Port=3
  Output2 : Outport  Port=4
  wires:
  Unit Delay/1 -> Output/1
  Unit Delay1/1 -> Output2/1, Scope/2
  In1/1 -> Unit Delay/1, Out1/1
  In2/1 -> Scope/1, Output1/1, Unit Delay1/1

== system controller14/State filters/Subsystem4/If Action Subsystem ==
  In1 : Inport
  In2 : Inport  Port=2
  Action Port : ActionPort  ActionPortLabel=else
  Divide : Product  Inputs=*/
  Out1 : Outport
  wires:
  In1/1 -> Divide/1
  In2/1 -> Divide/2
  Divide/1 -> Out1/1

== system controller14/State filters/Subsystem4/If Action Subsystem1 ==
  Action Port : ActionPort  ActionPortLabel=if(u1 == 0)
  Constant : Constant  Value=[0;0;0]
  Out1 : Outport
  wires:
  Constant/1 -> Out1/1

== system controller14/State filters/Subsystem4/Triggered Subsystem ==
  In1 : Inport
  In2 : Inport  Port=2
  Trigger : TriggerPort  VariantControl=(inherit)
  Scope : Scope  Commented=on  NumInputPorts=2
  Unit Delay : UnitDelay  SampleTime=-1  HasFrameUpgradeWarning=on
  Unit Delay1 : UnitDelay  SampleTime=-1  HasFrameUpgradeWarning=on
  Out1 : Outport
  Output : Outport  Port=2
  Output1 : Outport  Port=3
  Output2 : Outport  Port=4
  wires:
  Unit Delay/1 -> Output/1
  Unit Delay1/1 -> Output2/1, Scope/2
  In1/1 -> Unit Delay/1, Out1/1
  In2/1 -> Scope/1, Output1/1, Unit Delay1/1

== system controller14/State filters/Subsystem5/If Action Subsystem ==
  In1 : Inport
  In2 : Inport  Port=2
  Action Port : ActionPort  ActionPortLabel=else
  Divide : Product  Inputs=*/
  Out1 : Outport
  wires:
  In1/1 -> Divide/1
  In2/1 -> Divide/2
  Divide/1 -> Out1/1

== system controller14/State filters/Subsystem5/If Action Subsystem1 ==
  Action Port : ActionPort  ActionPortLabel=if(u1 == 0)
  Constant : Constant  Value=zeros(9,1)
  Out1 : Outport
  wires:
  Constant/1 -> Out1/1

== system controller14/State filters/Subsystem5/Triggered Subsystem ==
  R : Inport
  In2 : Inport  Port=2
  Trigger : TriggerPort  VariantControl=(inherit)
  Scope : Scope  Commented=on  NumInputPorts=2
  Unit Delay : UnitDelay  SampleTime=-1  HasFrameUpgradeWarning=on
  Unit Delay1 : UnitDelay  SampleTime=-1  HasFrameUpgradeWarning=on
  Out1 : Outport
  Output : Outport  Port=2
  Output1 : Outport  Port=3
  Output2 : Outport  Port=4
  wires:
  Unit Delay/1 -> Output/1
  Unit Delay1/1 -> Scope/2, Output2/1
  R/1 -> Unit Delay/1, Out1/1
  In2/1 -> Unit Delay1/1, Scope/1, Output1/1

== system controller14/signal generator1/Bias_Signal/AveragedBias ==
  note: To avoid having signal "jump",
      | we want SMOOTH transitions
      | in frequency (i.e., a weighted sum
      | of current freq and freq some delta t ago)
  note: time constant = 0.002sec
  In1 : Inport
  Discrete Transfer Fcn : DiscreteTransferFcn  Commented=through  Numerator=[0.05]  Denominator=[1 -.95]
  Out1 : Outport
  wires:
  In1/1 -> Discrete Transfer Fcn/1
  Discrete Transfer Fcn/1 -> Out1/1

== system controller14/signal generator1/Bias_Signal/SIgnalForRamp_binary ==
  note: Should output 1 or -1,
      | so signal ramps UP to 1
      | or DOWN to 0.
  In1 : Inport
  Add : Sum  Inputs=+-
  Compare To Zero : simulink/Logic and Bit Operations/Compare To Zero  relop=>  OutDataTypeStr=uint8  ZeroCross=off
  Constant : Constant
  Data Type Conversion : DataTypeConversion  OutDataTypeStr=double  SaturateOnIntegerOverflow=off  RndMeth=Floor
  Gain : Gain  Gain=2
  Out1 : Outport
  wires:
  In1/1 -> Compare To Zero/1
  Compare To Zero/1 -> Data Type Conversion/1
  Gain/1 -> Add/1
  Constant/1 -> Add/2
  Add/1 -> Out1/1
  Data Type Conversion/1 -> Gain/1

== system controller14/signal generator1/Drive_Signal1/AveragedAmp_filtered ==
  note: To avoid having signal "jump",
      | we want SMOOTH transitions
      | in frequency (i.e., a weighted sum
      | of current freq and freq some delta t ago)
  note: time constant 0.002sec
      | for 10kHz samping
  In1 : Inport
  Discrete Transfer Fcn : DiscreteTransferFcn  Commented=through  Numerator=[0.05]  Denominator=[1 -.95]
  Out1 : Outport
  wires:
  In1/1 -> Discrete Transfer Fcn/1
  Discrete Transfer Fcn/1 -> Out1/1

== system controller14/signal generator1/Drive_Signal1/AveragedOffset_filtered ==
  note: To avoid having signal "jump",
      | we want SMOOTH transitions
      | in frequency (i.e., a weighted sum
      | of current freq and freq some delta t ago)
  note: c
  note: time constant 0.02sec
      | for 10kHz samping
  In1 : Inport
  Discrete Transfer Fcn : DiscreteTransferFcn  Commented=through  Numerator=[0.05]  Denominator=[1 -.95]
  Out1 : Outport
  wires:
  In1/1 -> Discrete Transfer Fcn/1
  Discrete Transfer Fcn/1 -> Out1/1

== system controller14/signal generator1/Drive_Signal1/AveragedTau_filtered ==
  note: To avoid having signal "jump",
      | we want SMOOTH transitions
      | in frequency (i.e., a weighted sum
      | of current freq and freq some delta t ago)
  note: time constant 0.002sec
      | for 10kHz samping
  In1 : Inport
  Discrete Transfer Fcn : DiscreteTransferFcn  Numerator=[0.05]  Denominator=[1, -0.95]
  Out1 : Outport
  wires:
  In1/1 -> Discrete Transfer Fcn/1
  Discrete Transfer Fcn/1 -> Out1/1

== system controller14/signal generator1/Drive_Signal1/SignalForRamp_binary ==
  note: Should output 1 or -1,
      | so signal ramps UP to 1
      | or DOWN to 0.
  In1 : Inport
  Add : Sum  Inputs=+-
  Compare To Zero : simulink/Logic and Bit Operations/Compare To Zero  relop=>  OutDataTypeStr=uint8  ZeroCross=off
  Constant : Constant
  Data Type Conversion : DataTypeConversion  OutDataTypeStr=double  SaturateOnIntegerOverflow=off  RndMeth=Floor
  Gain : Gain  Gain=2
  Out1 : Outport
  wires:
  In1/1 -> Compare To Zero/1
  Compare To Zero/1 -> Data Type Conversion/1
  Gain/1 -> Add/1
  Constant/1 -> Add/2
  Add/1 -> Out1/1
  Data Type Conversion/1 -> Gain/1

== system controller14/signal generator1/Drive_Signal1/SignalForSin_binary ==
  note: We want this to stay "high" for 1
      | second after the actual "enable"
      | is turned off...
  In1 : Inport
  Compare To Zero : simulink/Logic and Bit Operations/Compare To Zero  relop=>  OutDataTypeStr=uint8  ZeroCross=off
  Data Type Conversion : DataTypeConversion  OutDataTypeStr=double  SaturateOnIntegerOverflow=off  RndMeth=Floor
  Out1 : Outport
  wires:
  In1/1 -> Compare To Zero/1
  Compare To Zero/1 -> Data Type Conversion/1
  Data Type Conversion/1 -> Out1/1

== system controller14/signal generator1/Drive_Signal1/Subsystem ==
  note: positive value pushes the left wing forward
  split cycle mu : Inport
  In2 : Inport  Port=2
  1-mu : Sum  Inputs=+-
  2f : Gain  Gain=2
  2nd harmonic : Trigonometry  OutputSignalType=real
  2pi : Gain  Gain=2*pi
  Abs1 : Abs  SaturateOnIntegerOverflow=off
  Add : Sum
  Constant : Constant
  combined sines : Sum
  deg to rad : Gain  Gain=pi/180
  f : Gain  Gain=-1
  first harmonic : Trigonometry  OutputSignalType=real
  omega*t : DiscreteIntegrator  SampleTime=-1  ICPrevOutput=DiscIntNeverNeededParam  ICPrevScaledInput=DiscIntNeverNeededParam
  phase offset : Constant  Value=0
  signal with gain1 : Product  RndMeth=Zero
  signal with gain2 : Product  RndMeth=Zero
  split cycle signal : Outport
  wires:
  2f/1 -> 2nd harmonic/1
  first harmonic/1 -> signal with gain1/2
  Constant/1 -> 1-mu/1
  split cycle mu/1 -> f/1, Abs1/1
  1-mu/1 -> signal with gain1/1
  2nd harmonic/1 -> signal with gain2/2
  signal with gain1/1 -> combined sines/1
  signal with gain2/1 -> combined sines/2
  combined sines/1 -> split cycle signal/1
  f/1 -> signal with gain2/1
  Abs1/1 -> 1-mu/2
  In2/1 -> 2pi/1
  2pi/1 -> omega*t/1
  omega*t/1 -> Add/2
  Add/1 -> first harmonic/1, 2f/1
  phase offset/1 -> deg to rad/1
  deg to rad/1 -> Add/1

== system controller14/signal generator1/Drive_Signal2/AveragedAmp_filtered ==
  note: To avoid having signal "jump",
      | we want SMOOTH transitions
      | in frequency (i.e., a weighted sum
      | of current freq and freq some delta t ago)
  note: time constant 0.002sec
      | for 10kHz samping
  In1 : Inport
  Discrete Transfer Fcn : DiscreteTransferFcn  Numerator=[0.05]  Denominator=[1 -.95]
  Out1 : Outport
  wires:
  In1/1 -> Discrete Transfer Fcn/1
  Discrete Transfer Fcn/1 -> Out1/1

== system controller14/signal generator1/Drive_Signal2/AveragedOffset_filtered ==
  note: To avoid having signal "jump",
      | we want SMOOTH transitions
      | in frequency (i.e., a weighted sum
      | of current freq and freq some delta t ago)
  note: c
  note: time constant 0.02sec
      | for 10kHz samping
  In1 : Inport
  Discrete Transfer Fcn : DiscreteTransferFcn  Numerator=[0.05]  Denominator=[1 -.95]
  Out1 : Outport
  wires:
  In1/1 -> Discrete Transfer Fcn/1
  Discrete Transfer Fcn/1 -> Out1/1

== system controller14/signal generator1/Drive_Signal2/AveragedTau_filtered ==
  note: To avoid having signal "jump",
      | we want SMOOTH transitions
      | in frequency (i.e., a weighted sum
      | of current freq and freq some delta t ago)
  note: time constant 0.002sec
      | for 10kHz samping
  In1 : Inport
  Discrete Transfer Fcn : DiscreteTransferFcn  Numerator=[0.05]  Denominator=[1, -0.95]
  Out1 : Outport
  wires:
  In1/1 -> Discrete Transfer Fcn/1
  Discrete Transfer Fcn/1 -> Out1/1

== system controller14/signal generator1/Drive_Signal2/SignalForRamp_binary ==
  note: Should output 1 or -1,
      | so signal ramps UP to 1
      | or DOWN to 0.
  In1 : Inport
  Add : Sum  Inputs=+-
  Compare To Zero : simulink/Logic and Bit Operations/Compare To Zero  relop=>  OutDataTypeStr=uint8  ZeroCross=off
  Constant : Constant
  Data Type Conversion : DataTypeConversion  OutDataTypeStr=double  SaturateOnIntegerOverflow=off  RndMeth=Floor
  Gain : Gain  Gain=2
  Out1 : Outport
  wires:
  In1/1 -> Compare To Zero/1
  Compare To Zero/1 -> Data Type Conversion/1
  Gain/1 -> Add/1
  Constant/1 -> Add/2
  Add/1 -> Out1/1
  Data Type Conversion/1 -> Gain/1

== system controller14/signal generator1/Drive_Signal2/SignalForSin_binary ==
  note: We want this to stay "high" for 1
      | second after the actual "enable"
      | is turned off...
  In1 : Inport
  Compare To Zero : simulink/Logic and Bit Operations/Compare To Zero  relop=>  OutDataTypeStr=uint8  ZeroCross=off
  Data Type Conversion : DataTypeConversion  OutDataTypeStr=double  SaturateOnIntegerOverflow=off  RndMeth=Floor
  Out1 : Outport
  wires:
  In1/1 -> Compare To Zero/1
  Compare To Zero/1 -> Data Type Conversion/1
  Data Type Conversion/1 -> Out1/1

== system controller14/signal generator1/Drive_Signal2/Subsystem ==
  note: positive value pushes the left wing forward
  split cycle mu : Inport
  In2 : Inport  Port=2
  1-mu : Sum  Inputs=+-
  2f : Gain  Gain=2
  2nd harmonic : Trigonometry  OutputSignalType=real
  2pi : Gain  Gain=2*pi
  Abs1 : Abs  SaturateOnIntegerOverflow=off
  Add : Sum
  Constant : Constant
  combined sines : Sum
  deg to rad : Gain  Gain=pi/180
  f : Gain  Gain=-1
  first harmonic : Trigonometry  OutputSignalType=real
  omega*t : DiscreteIntegrator  SampleTime=-1  ICPrevOutput=DiscIntNeverNeededParam  ICPrevScaledInput=DiscIntNeverNeededParam
  phase offset : Constant  Value=0
  signal with gain1 : Product  RndMeth=Zero
  signal with gain2 : Product  RndMeth=Zero
  split cycle signal : Outport
  wires:
  2f/1 -> 2nd harmonic/1
  first harmonic/1 -> signal with gain1/2
  Constant/1 -> 1-mu/1
  split cycle mu/1 -> f/1, Abs1/1
  1-mu/1 -> signal with gain1/1
  2nd harmonic/1 -> signal with gain2/2
  signal with gain1/1 -> combined sines/1
  signal with gain2/1 -> combined sines/2
  combined sines/1 -> split cycle signal/1
  f/1 -> signal with gain2/1
  Abs1/1 -> 1-mu/2
  In2/1 -> 2pi/1
  2pi/1 -> omega*t/1
  omega*t/1 -> Add/2
  Add/1 -> first harmonic/1, 2f/1
  phase offset/1 -> deg to rad/1
  deg to rad/1 -> Add/1

== system controller14/signal generator1/Drive_Signal3/AveragedAmp_filtered ==
  note: To avoid having signal "jump",
      | we want SMOOTH transitions
      | in frequency (i.e., a weighted sum
      | of current freq and freq some delta t ago)
  note: time constant 0.002sec
      | for 10kHz samping
  In1 : Inport
  Discrete Transfer Fcn : DiscreteTransferFcn  Numerator=[0.05]  Denominator=[1 -.95]
  Out1 : Outport
  wires:
  In1/1 -> Discrete Transfer Fcn/1
  Discrete Transfer Fcn/1 -> Out1/1

== system controller14/signal generator1/Drive_Signal3/AveragedOffset_filtered ==
  note: To avoid having signal "jump",
      | we want SMOOTH transitions
      | in frequency (i.e., a weighted sum
      | of current freq and freq some delta t ago)
  note: c
  note: time constant 0.02sec
      | for 10kHz samping
  In1 : Inport
  Discrete Transfer Fcn : DiscreteTransferFcn  Numerator=[0.05]  Denominator=[1 -.95]
  Out1 : Outport
  wires:
  In1/1 -> Discrete Transfer Fcn/1
  Discrete Transfer Fcn/1 -> Out1/1

== system controller14/signal generator1/Drive_Signal3/AveragedTau_filtered ==
  note: To avoid having signal "jump",
      | we want SMOOTH transitions
      | in frequency (i.e., a weighted sum
      | of current freq and freq some delta t ago)
  note: time constant 0.002sec
      | for 10kHz samping
  In1 : Inport
  Discrete Transfer Fcn : DiscreteTransferFcn  Numerator=[0.05]  Denominator=[1 -.95]
  Out1 : Outport
  wires:
  In1/1 -> Discrete Transfer Fcn/1
  Discrete Transfer Fcn/1 -> Out1/1

== system controller14/signal generator1/Drive_Signal3/SignalForRamp_binary ==
  note: Should output 1 or -1,
      | so signal ramps UP to 1
      | or DOWN to 0.
  In1 : Inport
  Add : Sum  Inputs=+-
  Compare To Zero : simulink/Logic and Bit Operations/Compare To Zero  relop=>  OutDataTypeStr=uint8  ZeroCross=off
  Constant : Constant
  Data Type Conversion : DataTypeConversion  OutDataTypeStr=double  SaturateOnIntegerOverflow=off  RndMeth=Floor
  Gain : Gain  Gain=2
  Out1 : Outport
  wires:
  In1/1 -> Compare To Zero/1
  Compare To Zero/1 -> Data Type Conversion/1
  Gain/1 -> Add/1
  Constant/1 -> Add/2
  Add/1 -> Out1/1
  Data Type Conversion/1 -> Gain/1

== system controller14/signal generator1/Drive_Signal3/SignalForSin_binary ==
  note: We want this to stay "high" for 1
      | second after the actual "enable"
      | is turned off...
  In1 : Inport
  Compare To Zero : simulink/Logic and Bit Operations/Compare To Zero  relop=>  OutDataTypeStr=uint8  ZeroCross=off
  Data Type Conversion : DataTypeConversion  OutDataTypeStr=double  SaturateOnIntegerOverflow=off  RndMeth=Floor
  Out1 : Outport
  wires:
  In1/1 -> Compare To Zero/1
  Compare To Zero/1 -> Data Type Conversion/1
  Data Type Conversion/1 -> Out1/1

== system controller14/signal generator1/Drive_Signal3/Subsystem ==
  split cycle mu : Inport
  In2 : Inport  Port=2
  1-mu : Sum  Inputs=+-
  2f : Gain  Gain=2
  2nd harmonic : Trigonometry  OutputSignalType=real
  2pi : Gain  Gain=2*pi
  Abs1 : Abs  SaturateOnIntegerOverflow=off
  Constant : Constant
  SmoothClock : DiscreteIntegrator  SampleTime=-1  ICPrevOutput=DiscIntNeverNeededParam  ICPrevScaledInput=DiscIntNeverNeededParam
  combined sines : Sum
  f : Gain
  first harmonic : Trigonometry  OutputSignalType=real
  signal with gain1 : Product  RndMeth=Zero
  signal with gain2 : Product  RndMeth=Zero
  split cycle signal : Outport
  wires:
  SmoothClock/1 -> first harmonic/1, 2f/1
  2f/1 -> 2nd harmonic/1
  2pi/1 -> SmoothClock/1
  first harmonic/1 -> signal with gain1/2
  Constant/1 -> 1-mu/1
  split cycle mu/1 -> f/1, Abs1/1
  1-mu/1 -> signal with gain1/1
  2nd harmonic/1 -> signal with gain2/2
  signal with gain1/1 -> combined sines/1
  signal with gain2/1 -> combined sines/2
  combined sines/1 -> split cycle signal/1
  In2/1 -> 2pi/1
  f/1 -> signal with gain2/1
  Abs1/1 -> 1-mu/2

== system controller14/signal generator1/Drive_Signal4/AveragedAmp_filtered ==
  note: To avoid having signal "jump",
      | we want SMOOTH transitions
      | in frequency (i.e., a weighted sum
      | of current freq and freq some delta t ago)
  note: time constant 0.002sec
      | for 10kHz samping
  In1 : Inport
  Discrete Transfer Fcn : DiscreteTransferFcn  Commented=through  Numerator=[0.05]  Denominator=[1 -.95]
  Out1 : Outport
  wires:
  In1/1 -> Discrete Transfer Fcn/1
  Discrete Transfer Fcn/1 -> Out1/1

== system controller14/signal generator1/Drive_Signal4/AveragedOffset_filtered ==
  note: To avoid having signal "jump",
      | we want SMOOTH transitions
      | in frequency (i.e., a weighted sum
      | of current freq and freq some delta t ago)
  note: c
  note: time constant 0.02sec
      | for 10kHz samping
  In1 : Inport
  Discrete Transfer Fcn : DiscreteTransferFcn  Commented=through  Numerator=[0.05]  Denominator=[1 -.95]
  Out1 : Outport
  wires:
  In1/1 -> Discrete Transfer Fcn/1
  Discrete Transfer Fcn/1 -> Out1/1

== system controller14/signal generator1/Drive_Signal4/AveragedTau_filtered ==
  note: To avoid having signal "jump",
      | we want SMOOTH transitions
      | in frequency (i.e., a weighted sum
      | of current freq and freq some delta t ago)
  note: time constant 0.002sec
      | for 10kHz samping
  In1 : Inport
  Discrete Transfer Fcn : DiscreteTransferFcn  Numerator=[0.05]  Denominator=[1, -0.95]
  Out1 : Outport
  wires:
  In1/1 -> Discrete Transfer Fcn/1
  Discrete Transfer Fcn/1 -> Out1/1

== system controller14/signal generator1/Drive_Signal4/SignalForRamp_binary ==
  note: Should output 1 or -1,
      | so signal ramps UP to 1
      | or DOWN to 0.
  In1 : Inport
  Add : Sum  Inputs=+-
  Compare To Zero : simulink/Logic and Bit Operations/Compare To Zero  relop=>  OutDataTypeStr=uint8  ZeroCross=off
  Constant : Constant
  Data Type Conversion : DataTypeConversion  OutDataTypeStr=double  SaturateOnIntegerOverflow=off  RndMeth=Floor
  Gain : Gain  Gain=2
  Out1 : Outport
  wires:
  In1/1 -> Compare To Zero/1
  Compare To Zero/1 -> Data Type Conversion/1
  Gain/1 -> Add/1
  Constant/1 -> Add/2
  Add/1 -> Out1/1
  Data Type Conversion/1 -> Gain/1
